simulink library "sun_point_SP_power_lib"  (R2016b)
settings: Solver=VariableStepAuto  StartTime=0.0  StopTime=10.0  RelTol=1e-3
undefined symbols (not defined in the file or in its folder): fsw_params
libraries: dspmathops x3, aerolibutil x1, ss_vec_2_angles x1
settings Model: Creator=taylorreynolds  LastModifiedBy=taylorreynolds

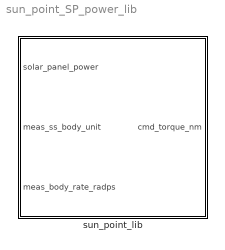
== system sun_point_SP_power_lib ==
  sun_point_lib : Subsystem  TreatAsAtomicUnit=on
      settings: MinAlgLoopOccurrences=on  RTWFcnNameOpts=Use subsystem name  RTWFileNameOpts=Use subsystem name

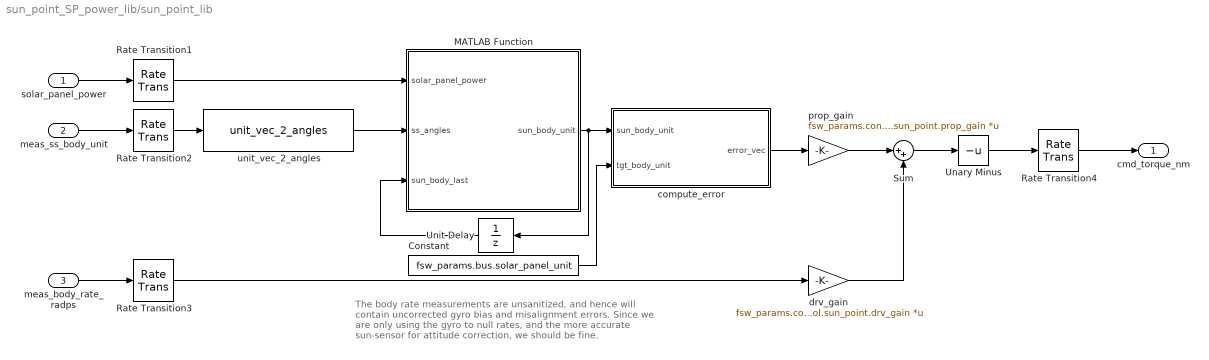
== system sun_point_SP_power_lib/sun_point_lib ==
  note: The body rate measurements are unsanitized, and hence will contain
      | uncorrected gyro bias and misalignment errors. Since we are only using
      | the gyro to null rates, and the more accurate sun-sensor for attitude
      | correction, we should be fine.
  solar_panel_power : Inport
  meas_ss_body_unit : Inport  Port=2
  meas_body_rate_radps : Inport  Port=3
  Constant : Constant  Value=fsw_params.bus.solar_panel_unit
  MATLAB Function : MATLAB Function  TreatAsAtomicUnit=on
  Rate Transition1 : RateTransition  X0=fsw_params.control.sun_point.ic.meas_pd_body_unit  OutPortSampleTime=fsw_params.control.sun_point.sample_time_s
  Rate Transition2 : RateTransition  X0=fsw_params.control.sun_point.ic.meas_ss_body_unit  OutPortSampleTime=fsw_params.control.sun_point.sample_time_s
  Rate Transition3 : RateTransition  X0=fsw_params.control.sun_point.ic.meas_body_rate_radps  OutPortSampleTime=fsw_params.control.sun_point.sample_time_s
  Rate Transition4 : RateTransition  X0=fsw_params.control.sun_point.ic.cmd_torque_nm  OutPortSampleTimeOpt=Inherit
  Sum : Sum  Inputs=|++
  Unary Minus : UnaryMinus
  Unit Delay : UnitDelay  InitialCondition=[1;0;0]  SampleTime=-1
  compute_error : Subsystem
  drv_gain : Gain  Gain=fsw_params.control.sun_point.drv_gain  Multiplication=Matrix(K*u)
  prop_gain : Gain  Gain=fsw_params.control.sun_point.prop_gain  Multiplication=Matrix(K*u)
  unit_vec_2_angles : ss_vec_2_angles/unit_vec_2_angles
  cmd_torque_nm : Outport
  wires:
  drv_gain/1 -> Sum/2
  Unit Delay/1 -> MATLAB Function/3(sun_body_last)
  Rate Transition4/1 -> cmd_torque_nm/1
  Unary Minus/1 -> Rate Transition4/1
  Sum/1 -> Unary Minus/1
  meas_body_rate_radps/1 -> Rate Transition3/1
  prop_gain/1 -> Sum/1
  meas_ss_body_unit/1 -> Rate Transition2/1
  Constant/1 -> compute_error/2(tgt_body_unit)
  Rate Transition2/1 -> unit_vec_2_angles/1
  compute_error/1(error_vec) -> prop_gain/1
  solar_panel_power/1 -> Rate Transition1/1
  Rate Transition3/1 -> drv_gain/1
  Rate Transition1/1 -> MATLAB Function/1(solar_panel_power)
  MATLAB Function/1(sun_body_unit) -> compute_error/1(sun_body_unit), Unit Delay/1
  unit_vec_2_angles/1 -> MATLAB Function/2(ss_angles)

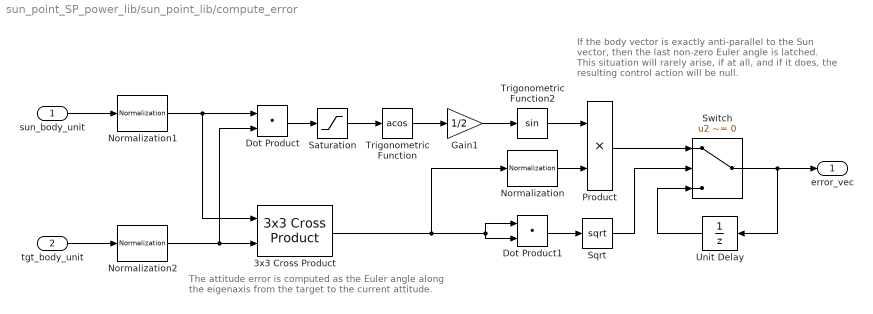
== system sun_point_SP_power_lib/sun_point_lib/compute_error ==
  note: The attitude error is computed as the Euler angle along the
      | eigenaxis from the target to the current attitude.
  note: If the body vector is exactly anti-parallel to the Sun vector,
      | then the last non-zero Euler angle is latched. This situation
      | will rarely arise, if at all, and if it does, the resulting
      | control action will be null.
  sun_body_unit : Inport
  tgt_body_unit : Inport  Port=2
  3x3 Cross Product : aerolibutil/3x3 Cross Product
  Dot Product : DotProduct  InputSameDT=on  OutDataTypeStr=Inherit: Inherit via internal rule
  Dot Product1 : DotProduct  InputSameDT=on  OutDataTypeStr=Inherit: Inherit via internal rule
  Gain1 : Gain  Gain=1/2
  Normalization : dspmathops/Normalization  NormType=2-norm  Bias=1e-10  NormOver=Each column  Dimension=1  outputDataTypeStr=Inherit: Same as product output  outputLastDataTypeStr=Inherit: Same as product output  outputMin=[]  outputMax=[]  accumDataTypeStr=Inherit: Same as product output  accumLastDataTypeStr=Inherit: Same as product output  roundingMode=Floor  overflowMode=off
  Normalization1 : dspmathops/Normalization  NormType=2-norm  Bias=1e-10  NormOver=Each column  Dimension=1  outputDataTypeStr=Inherit: Same as product output  outputLastDataTypeStr=Inherit: Same as product output  outputMin=[]  outputMax=[]  accumDataTypeStr=Inherit: Same as product output  accumLastDataTypeStr=Inherit: Same as product output  roundingMode=Floor  overflowMode=off
  Normalization2 : dspmathops/Normalization  NormType=2-norm  Bias=1e-10  NormOver=Each column  Dimension=1  outputDataTypeStr=Inherit: Same as product output  outputLastDataTypeStr=Inherit: Same as product output  outputMin=[]  outputMax=[]  accumDataTypeStr=Inherit: Same as product output  accumLastDataTypeStr=Inherit: Same as product output  roundingMode=Floor  overflowMode=off
  Product : Product
  Saturation : Saturate  UpperLimit=1  LowerLimit=-1
      settings: AttributesFormatString=|
      | U: %<UpperLimit>
      | L: %<LowerLimit>
  Sqrt : Sqrt  SaturateOnIntegerOverflow=on
  Switch : Switch  Criteria=u2 ~= 0
  Trigonometric Function : Trigonometry  Operator=acos
  Trigonometric Function2 : Trigonometry
  Unit Delay : UnitDelay  InitialCondition=fsw_params.control.sun_point.ic.error_vec  SampleTime=-1
  error_vec : Outport
  wires:
  Normalization2/1 -> 3x3 Cross Product/2, Dot Product/2
  Normalization1/1 -> Dot Product/1, 3x3 Cross Product/1
  3x3 Cross Product/1 -> Normalization/1, Dot Product1/1, Dot Product1/2
  Dot Product1/1 -> Sqrt/1
  Sqrt/1 -> Switch/2
  Unit Delay/1 -> Switch/3
  Switch/1 -> Unit Delay/1, error_vec/1
  Dot Product/1 -> Saturation/1
  Trigonometric Function/1 -> Gain1/1
  Normalization/1 -> Product/2
  Gain1/1 -> Trigonometric Function2/1
  Saturation/1 -> Trigonometric Function/1
  sun_body_unit/1 -> Normalization1/1
  Product/1 -> Switch/1
  Trigonometric Function2/1 -> Product/1
  tgt_body_unit/1 -> Normalization2/1

== matlab function sun_point_SP_power_lib/sun_point_lib/MATLAB Function ==
  data: solar_panel_power input size=3; sun_body_unit output size=3; ss_angles input size=2; sun_body_last input
function sun_body_unit = get_sun_body( solar_panel_power, ss_angles, sun_body_last )
% ----------------------------------------------------------------------- %
%GET_SUN_BODY   Estimates the unit vector pointing to the sun in the body
%frame based on the last valid sun sensor angles and the known solar panel
%power draws. 
%
% solar_panel_power is a 3x1 vector with +x in entry 1, -x in entry 2 and
% +y in entry 3.
%
%LOGIC: If any solar panels are generating sufficient power to claim the
%sun is hitting them, point that way. If none are, look at the last valid
%angle \alpha (about the x-axis) to decide between +/- z axis. Library
%never outputs +/- y axis, since the cross product with solar panel normal
%would return null.
%
% UW HuskySat-1, ADCS System
%
% T. Reynolds
% ----------------------------------------------------------------------- %

% Constants
tol         = 1e-3;
deg2rad     = pi/180;

% SS angles
alpha   = deg2rad * ss_angles(1);
beta    = deg2rad * ss_angles(2);

% Lower power thresholds [W]. Computed from P_max * 0.3 * (0.18/0.3), where
% first fraction is Earth's albedo, and second is the difference in
% efficiency for generating power from albedo vs. raw sunlight. From
% discussions with Sean Poulter, Power lead.
SP_Ptol_F   = 1.00; 
SP_Ptol_S   = 1.30;
sun_body_unit   = sun_body_last; % Choose arbitrary default value

[P,i] = max(solar_panel_power);
if( P - SP_Ptol_F > tol )
    if( (abs(i-1) < tol) && (abs(P - SP_Ptol_S) >= tol) )
        sun_body_unit  = [ 1; 0; 0 ];
    elseif( (abs(i-2) < tol) && (abs(P - SP_Ptol_S) >= tol) )
        sun_body_unit  = [ -1; 0; 0 ];
    elseif( (abs(i-3) < tol) && (abs(P - SP_Ptol_F) >= tol) )
        sun_body_unit  = rot_x(beta) * rot_y(alpha) *[ 0; 1; 0 ];
    end
else
    if( alpha > 0 )
        sun_body_unit = [ 0; 0; 1 ];
    else
        sun_body_unit = [ 0; 0; -1 ];
    end
end

end


function C = rot_x(s)
    C = [ 1 0 0; 0 cos(s) sin(s); 0 -sin(s) cos(s) ];
end

function C = rot_y(s)
    C = [ cos(s) 0 -sin(s); 0 1 0; sin(s) 0 cos(s) ];
end
